simulink model "Expriment_All2"  (R2014a)
settings: Solver=FixedStepDiscrete  SolverMode=SingleTasking  StartTime=0.0  StopTime=inf  FixedStep=0.01  RelTol=1e-3
PostLoadFcn:
  | h_RPStest = RPStest;
model workspace (MAT data in the model file):
  gtest = 0
undefined symbols (not defined in the file or in its folder): avert, avert_freq_factor, avert_gaze_dirs_chance, avert_gaze_duration_factor, avert_head_frequency_factor, avert_head_speed, BML, BML1, BML2, bmlsL, bmlsM, bodyBusyFlag, clock, emotion_amount_factor, faceBusyFlag, fileID, GAZE_WIN, gazing, mut_freq_factor, mutual_gaze_duration_factor, P, pose_cat_chance, pose_chanc_factor, pose_chance_factor, pose_frequency_factor, pose_lean, pose_lean_flag, pose_speed, pose_twitch, pr, serial, STATE_BEFORE, STATE_GO, STATE_OVER, STATE_READY, Stateflow
libraries: simulink x24, instrumentlib x6, lib_affectiveChar_behavior x2, realtime_pacer_lib x2, lib_affectiveChar_input x1
(part 3 of 7)

== matlab function Expriment_All2/facialExpr/facialExprGen/forloop1/displayBMLs ==
  data: e input; l input; i input double size=1 [1..]; bml input
function fcn(e,l,i,bml)
%#codegen
fprintf('%s','e:');fprintf('%f',e);
fprintf('%s','  ,L:');fprintf('%f',l);
fprintf('%s','  ,i:');fprintf('%f',i);
disp(decArr2Str(bml));

== matlab function Expriment_All2/facialExpr/facialExprGen/forloop1/makeBmls ==
  data: i input double size=1 [1..]; arrAU input; eAmount input; arrBML output
function arrBML = fcn(i,arrAU,eAmount)
    %#codegen
    coder.extrinsic('sprintf');
    coder.extrinsic('strcat');
    
    %Maryam, 14-10-2015
    %'strcat' dimension 2  maximum size is 453,it was not possible to concat and send all bmls 
    %for one emotion together(used simulink for loop )    
    
    AU=arrAU(i);eA=eAmount(i);   
    c1 = countDigits(AU);c2 = countDigits(eA);

    str1 = sprintf('<?xml version=\"1.0\" ?><act><bml>');
    
    if(max(ceil(log10(abs(AU))),1)==1) %if AU is one-digit
        temp = sprintf('<face type=\"FACS\" side=\"BOTH\" au=\"%1d\"  start=\"0\" ready=\"1\" stroke=\"2\"  relax=\"3\" end=\"4\" amount=\"%0.1f\"/>',AU,eA); 
        temp2=strcat(str1,temp);
        str1=temp2;
    else      
        temp = sprintf('<face type=\"FACS\" side=\"BOTH\" au=\"%2d\" start=\"0\" ready=\"1\" stroke=\"2\"  relax=\"3\" end=\"4\" amount=\"%0.1f\"/>',AU,eA);
        temp2=strcat(str1,temp);
        str1=temp2;
    end

    str2 = sprintf('</bml></act>');
    %n=length(arrAU);
    %mystr=blanks(arrAU(n));
    mystr=blanks(140+c1+c2);
    mystr = strcat (str1,str2);    
    arrBML = encStr2Arr(mystr);

== matlab function Expriment_All2/EmotionSubsystem/calculateValenceArousal/HELN_VA_Emo ==
  data: V input; e output double size=1; A input double
function e = fcn(V, A)

aVarTruthTableCondition_1 = false;
aVarTruthTableCondition_2 = false;
aVarTruthTableCondition_3 = false;
aVarTruthTableCondition_4 = false;
aVarTruthTableCondition_5 = false;
aVarTruthTableCondition_6 = false;
aVarTruthTableCondition_7 = false;
aVarTruthTableCondition_8 = false;


% 7-happy  2,1

aVarTruthTableCondition_1 = logical(V>10 && A<40 && A>10);

% 8-ex  1,2 AND 2,2

aVarTruthTableCondition_2 = logical(V>0 && A>40);

% 4-fear  -1,2 AND -2,2

aVarTruthTableCondition_3 = logical(V<0 && A>40);

% 3-frust  -2,1

aVarTruthTableCondition_4 = logical(V<-10 && A<40 && A>10);

% 6-idle  2,-1

aVarTruthTableCondition_5 = logical(V>10 && A<-10 && A>-40);

% 5-calm  1,-2 AND 2,-2

aVarTruthTableCondition_6 = logical(V>0 && A<-40);

% 1-bored  -1,-2 AND -2,-2

aVarTruthTableCondition_7 = logical(V<0 && A<-40);

% 2-sad  -2,-1

aVarTruthTableCondition_8 = logical(V<-10 && A<-10 && A>-40);

if (aVarTruthTableCondition_1)
    aFcnTruthTableAction_1();
elseif (aVarTruthTableCondition_2)
    aFcnTruthTableAction_2();
elseif (aVarTruthTableCondition_3)
    aFcnTruthTableAction_3();
elseif (aVarTruthTableCondition_4)
    aFcnTruthTableAction_4();
elseif (aVarTruthTableCondition_5)
    aFcnTruthTableAction_5();
elseif (aVarTruthTableCondition_6)
    aFcnTruthTableAction_6();
elseif (aVarTruthTableCondition_7)
    aFcnTruthTableAction_7();
elseif (aVarTruthTableCondition_8)
    aFcnTruthTableAction_8();
else % Default
    aFcnTruthTableAction_5();
end

function aFcnTruthTableAction_1()

% happy

e=7;

function aFcnTruthTableAction_2()

% excited

e=8;

function aFcnTruthTableAction_3()

% fear

e=4;

function aFcnTruthTableAction_4()

% frustration

e=3;

function aFcnTruthTableAction_5()

% idle

e=6;

function aFcnTruthTableAction_6()

% contempt

e=5;

function aFcnTruthTableAction_7()

% bored

e=1;

function aFcnTruthTableAction_8()

% sad

e=2;

== stateflow chart Expriment_All2/CharacterControl/personality_Behavior_Factors ==
  state setP
    entry:
    [mutual_gaze_duration_factor, avert_gaze_duration_factor,avert_head_frequency_factor,avert_head_speed,avert_gaze_dirs_chance,avert_freq_factor,mut_freq_factor,blink_flag, blinkperiod_min,blinkperiod_max]=sharedFunc.setGazeFactors(inV,inA,personality,personalityFlag,vaFlag,gazeArray,personalityChange);
    [pose_twitch,pose_frequency_factor,pose_chanc_factor,pose_cat_chance,pose_lean,pose_speed,pose_space,pose_lean_flag]=sharedFunc.setPoseFactors(inV,inA,personality,personalityFlag,vaFlag,poseArray,personalityChange);
  state init
    entry: mutual_gaze_duration_factor=1;avert_gaze_duration_factor=1;,avert_freq_factor=1;mut_freq_factor=1;
    avert_head_frequency_factor=20;avert_head_speed=1;avert_gaze_dirs_chance=1;blink_flag=0; blinkperiod_min=5;blinkperiod_max=9;
    pose_lean_flag=0; pose_frequency_factor=40;pose_chanc_factor=1;pose_cat_chance=50;pose_lean=18;pose_speed=1;pose_space=0;
  state wait
  state sharedFunc [group]
  (default) -> init
  init -> wait
  setP -> wait
  wait -> setP : [personalityChange==1]
  data: inA input double size=1; inV input double size=1; vaFlag input boolean size=1; personalityFlag input boolean size=1; gazeArray input double size=[1, 6]; personality input double size=1; personalityChange input boolean size=1; mutual_gaze_duration_factor data_store_memory; avert_head_frequency_factor data_store_memory; avert_gaze_duration_factor data_store_memory; avert_head_speed data_store_memory; avert_gaze_dirs_chance data_store_memory; poseArray input double size=[1, 6]; pose_chanc_factor data_store_memory; pose_frequency_factor data_store_memory; pose_lean data_store_memory; pose_change_flag data_store_memory; pose_lean_flag data_store_memory; pose_speed data_store_memory; pose_cat_chance data_store_memory; internalE input double size=1; emotion_amount_custom input double size=1; emotion_amount_factor data_store_memory size=1; mut_freq_factor data_store_memory; avert_freq_factor data_store_memory; pose_twitch data_store_memory; blinkperiod_min data_store_memory; blink_flag data_store_memory; blinkperiod_max data_store_memory; pose_space data_store_memory

== stateflow chart Expriment_All2/CharacterControl/custom_Behavior_Factors ==
  state setP
    entry:
    [mutual_gaze_duration_factor, avert_gaze_duration_factor,avert_head_frequency_factor,avert_head_speed,avert_gaze_dirs_chance,avert_freq_factor,mut_freq_factor]=sharedFunc.setGazeFactors(inV,inA,personality,personalityFlag,vaFlag,gazeArray,personalityChange);
  state init
    entry: mutual_gaze_duration_factor=1;avert_gaze_duration_factor=1;
    avert_head_frequency_factor=1;avert_head_speed=1;avert_gaze_dirs_chance=1;,avert_freq_factor=1;mut_freq_factor=1;
    pose_frequency_factor=5;pose_chanc_factor=1;pose_cat_chance=10;pose_lean=10;pose_speed=1;pose_lean_flag=0;
  state wait
  state sharedFunc [group]
  state setP1
    entry:
    [pose_twitch,pose_frequency_factor,pose_chanc_factor,pose_cat_chance,pose_lean,pose_speed,pose_lean_flag]=sharedFunc.setPoseFactors(inV,inA,personality,personalityFlag,vaFlag,poseArray,personalityChange);
  (default) -> init
  wait -> setP [order 1] : [gazeArray(:,1)==1]
  setP -> wait
  init -> wait
  setP1 -> wait
  wait -> setP1 [order 2] : [poseArray(:,1)==1]
  data: inA input double size=1; inV input double size=1; vaFlag input boolean size=1; personalityFlag input boolean size=1; gazeArray input double size=[1, 6]; personality input double size=1; personalityChange input boolean size=1; mutual_gaze_duration_factor data_store_memory; avert_head_frequency_factor data_store_memory; avert_gaze_duration_factor data_store_memory; avert_head_speed data_store_memory; avert_gaze_dirs_chance data_store_memory; poseArray input double size=[1, 6]; pose_lean data_store_memory; pose_speed data_store_memory; pose_chanc_factor data_store_memory; pose_frequency_factor data_store_memory; pose_cat_chance data_store_memory; pose_lean_flag data_store_memory; emotion_amount_custom input double size=1; emotion_amount_factor data_store_memory size=1; mut_freq_factor data_store_memory; avert_freq_factor data_store_memory; pose_twitch data_store_memory

== matlab function Expriment_All2/EmotionSubsystem/calculateValenceArousal/HELN plot ==
  data: v input; a input
function fcn(v,a)
%coder.extrinsic to bypass code generation
coder.extrinsic('fscanf')
coder.extrinsic('get_param');
% coder.extrinsic('importdata');

currentTime=get_param('Expriment_FacialExpr','SimulationTime');%use name of simulink proj

A = [v;a;currentTime];

fileID = fopen('HELN_VA_table.txt','a');
fprintf(fileID,'%0.1f,%0.1f,%0.1f\r\n',A);
fclose(fileID);

%use the following to draw the plot
%tmp_data = importdata('HEHN_VA_table.txt',','); 
%no need: x=tmp_data(:,1);y=tmp_data(:,2);z=tmp_data(:,3)
%matrix=tmp_data
%tri = delaunay(matrix(:,1),matrix(:,2));
%trisurf(tri,matrix(:,1),matrix(:,2),matrix(:,3))
%shading interp

%-----------------------------------------
% fileID = fopen('HEHN_VA_table.txt','r');
% formatSpec = '%1f\r %1f\r %1f\r\n';
% sizeA = [3 Inf];
% A = fscanf(fileID,formatSpec,sizeA)
% % A = A'
% fclose(fileID);

% x = zeros(100,2);y = zeros(100,2);
% filename = 'HEHN_VA_table.txt';
% delimiterIn = ' ';
% headerlinesIn = 1;
% A = importdata(filename,delimiterIn,headerlinesIn);

% fileID=fopen('HEHN_VA_table4.txt');
% s=textscan(fileID,'%d %d %d','headerlines',23);
% fclose(fileID);
% x=s{1}

== matlab function Expriment_All2/EmotionSubsystem/calculateValenceArousal/HEHN_V ==
  data: v2 output double size=1; v1 input double size=1
function v2 = fcn(v1)

aVarTruthTableCondition_1 = false;
aVarTruthTableCondition_2 = false;



aVarTruthTableCondition_1 = logical(v1>10);


aVarTruthTableCondition_2 = logical(v1<-10);

if (aVarTruthTableCondition_1)
    aFcnTruthTableAction_1();
elseif (aVarTruthTableCondition_2)
    aFcnTruthTableAction_2();
else % Default
    aFcnTruthTableAction_3();
end

function aFcnTruthTableAction_1()


v2=v1;

function aFcnTruthTableAction_2()


v2=v1;

function aFcnTruthTableAction_3()


v2=0;

== matlab function Expriment_All2/EmotionSubsystem/calculateValenceArousal/LEHN_V ==
  data: v2 output double size=1; v1 input double size=1
function v2 = fcn(v1)

aVarTruthTableCondition_1 = false;
aVarTruthTableCondition_2 = false;



aVarTruthTableCondition_1 = logical(v1>25);


aVarTruthTableCondition_2 = logical(v1<-25);

if (aVarTruthTableCondition_1)
    aFcnTruthTableAction_1();
elseif (aVarTruthTableCondition_2)
    aFcnTruthTableAction_2();
else % Default
    aFcnTruthTableAction_3();
end

function aFcnTruthTableAction_1()


v2=v1;

function aFcnTruthTableAction_2()


v2=v1;

function aFcnTruthTableAction_3()


v2=0;

== matlab function Expriment_All2/EmotionSubsystem/calculateValenceArousal/LELN_A ==
  data: a2 output double size=1; a1 input double size=1
function a2 = fcn(a1)

aVarTruthTableCondition_1 = false;
aVarTruthTableCondition_2 = false;



aVarTruthTableCondition_1 = logical(a1>25);


aVarTruthTableCondition_2 = logical(a1<-25);

if (aVarTruthTableCondition_1)
    aFcnTruthTableAction_1();
elseif (aVarTruthTableCondition_2)
    aFcnTruthTableAction_2();
else % Default
    aFcnTruthTableAction_3();
end

function aFcnTruthTableAction_1()


a2=a1;

function aFcnTruthTableAction_2()


a2=a1;

function aFcnTruthTableAction_3()


a2=0;

== matlab function Expriment_All2/EmotionSubsystem/calculateValenceArousal/LELN_VA_Emo ==
  data: V input; e output double size=1; A input double
function e = fcn(V, A)

aVarTruthTableCondition_1 = false;
aVarTruthTableCondition_2 = false;
aVarTruthTableCondition_3 = false;
aVarTruthTableCondition_4 = false;
aVarTruthTableCondition_5 = false;
aVarTruthTableCondition_6 = false;
aVarTruthTableCondition_7 = false;
aVarTruthTableCondition_8 = false;


% 7-happy  2,1

aVarTruthTableCondition_1 = logical(V>20 && A<40 && A>20);

% 8-ex  1,2 AND 2,2

aVarTruthTableCondition_2 = logical(V>0 && A>40);

% 4-fear  -1,2 AND -2,2

aVarTruthTableCondition_3 = logical(V<0 && A>40);

% 3-frust  -2,1

aVarTruthTableCondition_4 = logical(V<-20 && A<40 && A>20);

% 6-idle  2,-1

aVarTruthTableCondition_5 = logical(V>20 && A<-20 && A>-40);

% 5-calm  1,-2 AND 2,-2

aVarTruthTableCondition_6 = logical(V>0 && A<-40);

% 1-bored  -1,-2 AND -2,-2

aVarTruthTableCondition_7 = logical(V<0 && A<-40);

% 2-sad  -2,-1

aVarTruthTableCondition_8 = logical(V<-20 && A<-20 && A>-40);

if (aVarTruthTableCondition_1)
    aFcnTruthTableAction_1();
elseif (aVarTruthTableCondition_2)
    aFcnTruthTableAction_2();
elseif (aVarTruthTableCondition_3)
    aFcnTruthTableAction_3();
elseif (aVarTruthTableCondition_4)
    aFcnTruthTableAction_4();
elseif (aVarTruthTableCondition_5)
    aFcnTruthTableAction_5();
elseif (aVarTruthTableCondition_6)
    aFcnTruthTableAction_6();
elseif (aVarTruthTableCondition_7)
    aFcnTruthTableAction_7();
elseif (aVarTruthTableCondition_8)
    aFcnTruthTableAction_8();
else % Default
    aFcnTruthTableAction_5();
end

function aFcnTruthTableAction_1()

% happy

e=7;

function aFcnTruthTableAction_2()

% excited

e=8;

function aFcnTruthTableAction_3()

% fear

e=4;

function aFcnTruthTableAction_4()

% frustration

e=3;

function aFcnTruthTableAction_5()

% idle

e=6;

function aFcnTruthTableAction_6()

% contempt

e=5;

function aFcnTruthTableAction_7()

% bored

e=1;

function aFcnTruthTableAction_8()

% sad

e=2;

== matlab function Expriment_All2/EmotionSubsystem/satFunction ==
  data: randv input; smile input; wave input; win input; invade input; v_trigW output; vaFlag input; v_trig output
function [v_trigW,v_trig]= fcn(randv,smile,wave,win,invade,vaFlag)
%#codegen
% 30/06/2015
    %Here set Agent's satisfaction flag based on your scenario
    %In RPS scenario agent gets satisfined when she wins. states of interaction= {STATE_READY=7;
    %STATE_GO=1;STATE_HAND=2;STATE_OVER=3; STATE_BEFORE=4;STATE_RESULT=5;STATE_WAIT=6;}
   
    if(vaFlag==1)
        v_trigW=0;%weight by which valence value is changed (sum of weight of all triggers)
        %randv 30% chance of random increase or decrease in valence
        randTrigger=floor(randv);
        if(0<randTrigger)&&(randTrigger<30)
            v_trigW = v_trigW + 0.6;
        end
        if(30<randTrigger)&&(randTrigger<60)
            v_trigW = v_trigW - 0.6;
        end

        if(win==2) %agent wins so she is satisfied
            v_trigW = v_trigW + 0.5;
        elseif(win==1) %user wins so agent is NOT satisfied
            v_trigW = v_trigW - 0.5;
        end

        if(smile==1)
            v_trigW=v_trigW+0.25;
        end

        if(wave==1)
            v_trigW=v_trigW+0.25;
        end

        if(invade==1)
            v_trigW=v_trigW-0.25;
        end
    else
         v_trigW=0;
    end
    if(v_trigW>0)
        v_trig=1;
    elseif(v_trigW<0)
        v_trig=-1;
        v_trigW=abs(v_trigW);
    else
        v_trig=0;
    end

== matlab function Expriment_All2/CharacterControl/personality_Behavior_Factors/sharedFunc ==
  data: v function_input double size=1; a function_input double size=1; mutDurFactor function_output double size=1; avertDurFactor function_output double size=1; avertHeadFreqFactor function_output double size=1; p function_input double size=1; pFlag function_input boolean size=1; vaFlag function_input boolean size=1; avertHeadSpeed function_output double size=1; gazeArr function_input double size=[1,6]; avertDirsChance function_output double size=1; avertFreqFactor function_output double size=1; mutFreqFactor function_output double size=1; blinkFlag function_output double size=1; blinkPeriodMin function_output double size=1; blinkPeriodMax function_output double size=1; personalityChange function_input double size=1; poseTwitch function_output double size=1; poseFreqFactor function_output double size=1; poseChanceFactor function_output double size=1; poseCatChance function_output double size=1; poseLean function_output double size=1; v function_input double size=1; ar function_input double size=1; p function_input double size=1; pFlag function_input boolean size=1; vaFlag function_input boolean size=1; poseSpeed function_output double size=1; poseSpace function_output double size=1; poseArr function_input double size=[1,6]; poseLeanFlag function_output double size=1; personalityChange function_input double size=1
function [mutDurFactor,avertDurFactor,avertHeadFreqFactor,avertHeadSpeed,avertDirsChance,avertFreqFactor,mutFreqFactor,blinkFlag,blinkPeriodMin,blinkPeriodMax]=setGazeFactors(v,a,p,pFlag,vaFlag,gazeArr,personalityChange)
    % Valence/Arousal: ref?
    %V+A+ (excite,happy):high mutual dur,head avert freq less,high freq of change btw mut/avert(MMMMMMMAAMMMMMAMMMA)
    %V-A+ (fear,frust): mid mut/avert,,head avert freq mid,high freq of change btw mut/avert(MMAAMMMAAMMAAAMMMAAAMA)
    %V+A- (idle, calm): mid mut/avert,head avert freq mid,low freq of change btw mut/avert(MMMMMMMAAAAAAMMMMMAAAAA)
    %V-A- (bored,sad):  avert dur more,,head avert freq more,,high freq of change btw mut/avert(AAAAAAMAAAAAAAAMAAAAA)
    %V+A+: v>0 & a>0,V-A+: v<0 & a>0,V+A-:v>0 & a<0,V-A-:v<0 & a<0

    %paper: Effects of Direct and Averted Gaze on the Perception of Facially Communicated Emotion
    % rate of approach-oriented dispositions (i.e., anger and joy) higher for direct relative gaze stimuli
    %avoidance-oriented dispositions (i.e., fear and sadness) would be higher for averted gaze faces.

    %russel, mehrabian circumplex:
    % v-mid,a-mid:approach;     v-mid,a+:avoid;       v-mid,a-:avoid
    % v+,a-mid:mid-approach;    v+,a+:high-approach;  v+,a-:low-approach
    % v-,a-mid:mid-avoid;        v-,a+:high-avoid;    v-,a-:low-avoid

    % marsella, emotional gaze:
    % a+:high blink, faster move
    
    %PERSONALITY:
    % HEHN:mutual dur more,head avert freq more,high freq of change btw mut/avert(MAMAMMAMMMAMAMMAMMAMA)
    % LEHN:avert dur  more,head avert freq more, high freq of change btw mut/avert(AMAAMAAAMAMAAAMAAMAAM)
    % HELN:mutual dur  more,head avert freq less,low freq of change btw mut/avert(MMMMMMMAMMMMMMMMAMMM)
    % LELN:avert  dur more,head avert freq more,low freq of change btw mut/avert(AAAAAAMAAAAAAAAMAAAAA)
    
    %Perception of personality through eye gaze, Ruhland et al
    %Extravert: gaze tward,long,often,up-center-left-right; few blinks ; wide fast node
    %Introvert: gaze Avoidance,short,seldom,down-center; normal blinks; small slow node
    %Neurotic: gaze Avoidance,short,seldom,down-left-right; often blinks; None
    %Stable: gaze tward,medium,medium,center-left-right; normal blinks ; None
    
    %Saccadic reaction time is between 0.18sec and 0.22sec on average.Minimum intersaccadic interval ranges from 0.05sec to 0.1sec
    %smartbody DOF:magnitude:~btw 5'&12'->chanceO:btw 3&8->aveDur:btw 0.26sec&0.18sec --> 
    %simulation sample time is 0.001 so btw 26 and 18
    %magnitude=-6.9*log(chanceO/15.7) -->  -6.9*log(3/15.7)=11.4,-6.9*log(8/15.7)=4.6
    %chanceO=randArray(:,7)-->(3,8); 
    %avertDur=(25+2.5*magnitude)/2*factor;(same for mutual):btw(25+2.5*11.4)/2=26,(25+2.5*4.6)/2=18
    %randHeadChance=randi([1,1+round(randArray(3,5)/avert_head_frequency_factor)]);

    mutDurFactor=1; 
    avertDurFactor=1;  
    avertHeadFreqFactor=20;
    avertHeadSpeed=1;%1=normal, 2=fast&up,3=slow&down
    avertDirsChance=0;%not 1 & 2 is normal
    avertFreqFactor=1;
    mutFreqFactor=1;
    blinkFlag=0;
    blinkPeriodMin=5.0; %normal
    blinkPeriodMax=9.0;%normal

    if(pFlag==1)
        if(personalityChange==1)
            blinkFlag=1;disp('personality changed.');
        end
        if(p==1)%HEHN  
            mutDurFactor=2; % HEHN mut longer ,((25+2.5*magnitude)*mutual_gaze_duration_factor)/7;
            avertDurFactor=0.5;%HE avert short,3' to 4',btw (25+2.5*magnitude)*avert_gaze_duration_factor)/7;
            mutFreqFactor=4;%HE mut long,12' to 17'
            avertFreqFactor=0.25;% val/4, HE avert gaze low
            
            avertHeadFreqFactor=30;%HE often head,[avert_head_frequency_factor>randrandi(0,100)]
            avertHeadSpeed=2;%HE fast&up, headSpeed={1,2,3}
            avertDirsChance=1;%HE up            
            
            blinkPeriodMin=0.15; %HN often blinks
            blinkPeriodMax=6.0;%HE few blinks
        elseif(p==2) %LEHN %LE normal blinks, HN often blinks
            mutDurFactor=0.5; % LE mut less(mutDur/10) ,HN freq more
            avertDurFactor=2; % (avertDur/4)
            mutFreqFactor=0.15;
            avertFreqFactor=4;
            
            avertHeadFreqFactor=15;%LE avert low
            avertHeadSpeed=3;%LE slow&down
            avertDirsChance=2;%LE down
           
            blinkPeriodMin=0.2; %often
            blinkPeriodMax=5.0;%norm
        elseif(p==3) %HELN %HE few blinks, LN normal blinks 
            mutDurFactor=4; % HE dur more, LN freq less
            avertDurFactor=0.1; % /4 
            mutFreqFactor=4;
            avertFreqFactor=0.25;
            
            avertHeadFreqFactor=25;%HE avert head more
            avertHeadSpeed=2;%fast&up
            avertDirsChance=1;%HE up            
            
            blinkPeriodMin=5.0; %normal
            blinkPeriodMax=15.0;%few
        else %LELN %LE normal blinks, LN normal blinks 
            mutDurFactor=0.25; % /4 
            avertDurFactor=0.5;% /2 
            mutFreqFactor=0.25;
            avertFreqFactor=4;
            
            avertHeadFreqFactor=10;%LE avert head less
            avertHeadSpeed=3;%slow&down
            avertDirsChance=2;%LE down
          
            blinkPeriodMin=5.0; %normal
            blinkPeriodMax=9.0;%normal
        end  
    end
  
    %for emotion I should, seperate that from the controllers so they
    %calculate the depented parameters in parallel, in order to avoid a lot
    %of BMLs the checking state is repeating every 20 secs and if the value
    %is changed it sends the BML, here instead of constant value I should
    %make all of the parametric so when V & A increase or decrease it
    %affects the blink mut and avert ..
    if(vaFlag==1)
        if(v>40 && a>40)%V+A+,high-approach,mutual alot
            mutDurFactor=mutDurFactor*2; % /2
            avertDurFactor=round(avertDurFactor*0.5);  % /2
            avertHeadFreqFactor=round(avertHeadFreqFactor/3);%high-approach:head not avert
            %avertHeadSpeed=2;%aroused fast, removed ths since fast&up is together, also it makes it hard for evaluateion
            
            %27-12-2015- Best way to set the blink period is as a linear function of arousal amount
            %      val/(1+((2-1)*(A/100))) 
            %in which val is BlinkMin or BlinkMax and A is arousal amount; this function sets the
            %blinkPriodMin and max to half for twice blink in arousal=100 and to their default at 
            %arousal=1 sicne we need to re-calculate and send sbms continiously I avoided that for 
            % now, instead I only increase min and max when Arousal passes 50 threshold
            blinkPeriodMin=blinkPeriodMin/1.5; %often
            blinkPeriodMax=blinkPeriodMax/1.5;
            blinkFlag=1;
            disp(mutDurFactor);
        elseif(v<-40 && a>40) %V-A+,high-avoid, avert alot
            mutDurFactor=round(mutDurFactor*0.5); % /2
            avertDurFactor=avertDurFactor*2; % /2
            avertHeadFreqFactor=avertHeadFreqFactor+30;%high-avoid:head avert alot
            %avertHeadSpeed=2;%fast
            blinkPeriodMin=blinkPeriodMin/1.5; %often
            blinkPeriodMax=blinkPeriodMax/1.5;
            blinkFlag=1;
        elseif(v>40 && a<-40) %V+A- ,low-approach, mutual most
            mutDurFactor=round(mutDurFactor*1.5); %  /2
            avertDurFactor=round(avertDurFactor*0.75); %/2
            avertHeadFreqFactor=round(avertHeadFreqFactor/2);%approach:head not avert
            %avertHeadSpeed=1;%slow&down
            blinkFlag=0;
        elseif(v<-40 && a<-40) %V-A-,  low-avoid, avert most
            mutDurFactor=round(mutDurFactor*0.75); %/2
            avertDurFactor=round(avertDurFactor*1.5);% /2
            avertHeadFreqFactor=avertHeadFreqFactor+20;%avoid:head avert alot
            %avertHeadSpeed=1;%slow&down, if he is extrovert we dont want him to look down even if low aroused
            blinkFlag=0;
        end  
    end

== matlab function Expriment_All2/CharacterControl/personality_Behavior_Factors/sharedFunc ==
function [poseTwitch,poseFreqFactor,poseChanceFactor,poseCatChance,poseLean,poseSpeed,poseSpace,poseLeanFlag]=setPoseFactors(v,ar,p,pFlag,vaFlag,poseArr,personalityChange)   
    
    pose_custom_flag=poseArr(:,1);
    pose_chance_custom=poseArr(:,3);
    pose_selfAdaptor_chance_custom=poseArr(:,2);
    pose_frequency_custom=poseArr(:,4);
    pose_speed_custom=poseArr(:,5);
    pose_lean_custom=poseArr(:,6);

    poseCatChance=50;%defalut 50% chance of selfA or weightShift, due low num of weightShift
    poseChanceFactor=1;%if (not similar duration btw poses always)
    poseFreqFactor=40;
    poseSpeed=1;%1=normal;2=fast; 3=slow;
    poseLean=18;
    poseTwitch=0;
    poseLeanFlag=0;
    poseSpace=0;% normal people dont do spacious gestures

    if(pose_custom_flag==0)    
        if(pFlag==1)
            if(personalityChange==1)
                poseLeanFlag=1;
            end
            if(p==1) %HEHN
                 poseTwitch=1;%HN
                 poseFreqFactor=15;%HN more freq,after(pose_frequency_factor,secs)
                 poseLean=18;
                 poseChanceFactor=4;% HN high chance,randPoseChance=randi([0,round(interest*randSlowPose/pose_chance_factor)]);
                 poseCatChance=90;%HN high selfA,[randPR<=pose_selfAdaptor_chance_factor ]
                 poseSpeed=2;%HE fast
                 %poseSpace=1;%HE
             elseif(p==2)%LEHN
                 poseTwitch=1;%HN
                 poseFreqFactor=20;%HN more freq but low speed
                 poseLean=19;
                 poseChanceFactor=4;%HN high chance
                 poseCatChance=10;%HN high:90% adaptor
                 poseSpeed=3;%LE slow
                 %poseSpace=0;%LE
             elseif(p==3)%HELN
                 poseTwitch=0;%LN
                 poseFreqFactor=50;%LN low chance
                 poseLean=18;
                 poseChanceFactor=1;%LN low chance
                 poseCatChance=10;%  10% adapter
                 poseSpeed=2;%HE
                 %poseSpace=1;%HE
             elseif(p==4)%LELN
                 poseTwitch=0;%LN
                 poseFreqFactor=60;%LE
                 poseLean=19;
                 poseChanceFactor=1;%LN low chance
                 poseCatChance=90;
                 poseSpeed=3;%LE
                 %poseSpace=0;%LE
            else%no personality, its should not come here
                fprintf(' Error: the personality is not listed, back to normal, p=: '); fprintf('%0.0f',p);
                poseCatChance=70;
                poseChanceFactor=1;
                poseFreqFactor=40;
                poseSpeed=1;%1=normal;2=fast; 3=slow;
                poseLean=18;
                poseTwitch=0;
                poseLeanFlag=0;
                poseSpace=0;% normal people dont do spacious gestures
             end
        end
%     29-12-2015  I removed this since it intefere with personality's effect on pose
%     % marsella, emotional gaze:
%     % a+:faster move,body fw
%     if(vaFlag==1)
%         if( ar>50)%A+
%              poseSpeed=2;%high arouse fast move
%              poseLeanFlag=12;%high aroused lean fw
%         end
%         if(ar<-50)%A-
%              poseSpeed=3;%low arouse slow move
%              poseLeanFlag=11;%low aroused lean back
%         end
%     end 
    
    else%custom-flag==1
        poseFreqFactor=pose_frequency_custom;
        poseLean=pose_lean_custom;
        poseChanceFactor=pose_chance_custom;
        poseCatChance=pose_selfAdaptor_chance_custom;
        poseSpeed=pose_speed_custom;
    end

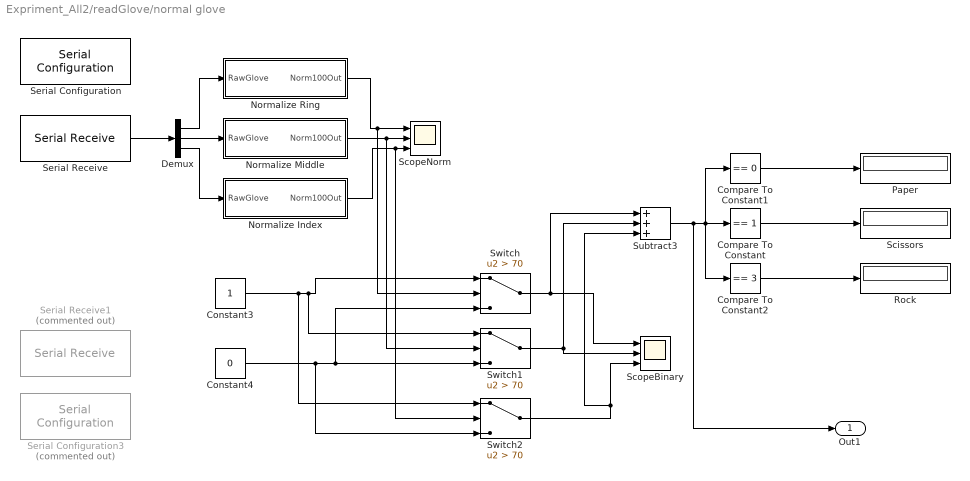
== system Expriment_All2/readGlove/normal glove ==
  Compare To Constant : simulink/Logic and Bit Operations/Compare To Constant  relop===  const=1  OutDataTypeStr=boolean
  Compare To Constant1 : simulink/Logic and Bit Operations/Compare To Constant  relop===  const=0  OutDataTypeStr=boolean
  Compare To Constant2 : simulink/Logic and Bit Operations/Compare To Constant  relop===  const=3  OutDataTypeStr=boolean
  Constant3 : Constant
  Constant4 : Constant  Value=0
  Demux : Demux  Outputs=3
  Normalize Index : Subsystem
  Normalize Middle : Subsystem
  Normalize Ring : Subsystem
  Paper : Display
  Rock : Display
  Scissors : Display
  ScopeBinary : Scope  NumInputPorts=3
      settings: YMin=-0.5~-0.5~-0.5  YMax=1.5~1.5~1.5
  ScopeNorm : Scope  NumInputPorts=3
      settings: TimeRange=10  YMin=-20~-20~-20  YMax=150~150~150
  Serial Configuration : instrumentlib/Serial Configuration  Priority=-200000  ComPortMenu=<Please select a port...>  ComPort=COM4  ObjConstructor=serial('COM4');  BaudRate=9600  DataBits=8  Parity=none  StopBits=1  FlowControl=none  Timeout=10  ByteOrder=LittleEndian
  Serial Configuration3 : instrumentlib/Serial Configuration  Priority=-200000  Commented=on  ComPortMenu=<Please select a port...>  ComPort=COM5  ObjConstructor=serial('COM5');  BaudRate=9600  DataBits=8  Parity=none  StopBits=1  FlowControl=none  Timeout=10  ByteOrder=LittleEndian
  Serial Receive : instrumentlib/Serial Receive  ComPortMenu=<Please select a port...>  ComPort=COM4  ObjConstructor=serial('COM4');  Terminator=<none>  DataSize="[3  1]"  DataType=uint8  EnableBlockingMode=on  ActionDataUnavailable=Output last received value  CustomValue=0  SampleTime=0.01
  Serial Receive1 : instrumentlib/Serial Receive  Commented=on  ComPortMenu=<Please select a port...>  ComPort=COM5  ObjConstructor=serial('COM5');  Terminator=<none>  DataSize="[3  1]"  DataType=uint8  EnableBlockingMode=on  ActionDataUnavailable=Output last received value  CustomValue=0  SampleTime=0.01
  Subtract3 : Sum  Inputs=+++
  Switch : Switch  Criteria=u2 > Threshold  Threshold=70
  Switch1 : Switch  Criteria=u2 > Threshold  Threshold=70
  Switch2 : Switch  Criteria=u2 > Threshold  Threshold=70
  Out1 : Outport
  wires:
  Demux/1 -> Normalize Ring/1(RawGlove)
  Demux/2 -> Normalize Middle/1(RawGlove)
  Demux/3 -> Normalize Index/1(RawGlove)
  Switch/1 -> ScopeBinary/1, Subtract3/1
  Constant3/1 -> Switch2/1, Switch1/1, Switch/1
  Constant4/1 -> Switch2/3, Switch1/3, Switch/3
  Switch1/1 -> ScopeBinary/2, Subtract3/2
  Switch2/1 -> Subtract3/3, ScopeBinary/3
  Subtract3/1 -> Compare To Constant/1, Compare To Constant2/1, Compare To Constant1/1, Out1/1
  Compare To Constant1/1 -> Paper/1
  Compare To Constant/1 -> Scissors/1
  Compare To Constant2/1 -> Rock/1
  Normalize Index/1(Norm100Out) -> Switch2/2, ScopeNorm/3
  Normalize Ring/1(Norm100Out) -> Switch/2, ScopeNorm/1
  Normalize Middle/1(Norm100Out) -> ScopeNorm/2, Switch1/2
  Serial Receive/1 -> Demux/1

== system Expriment_All2/readSHORE/smile ==
  In1 : Inport
  ifSmile : MATLAB Function  TreatAsAtomicUnit=on
  Out1 : Outport
  wires:
  ifSmile/1(y) -> Out1/1
  In1/1 -> ifSmile/1(u)

== system Expriment_All2/GazeFollowSubsystem/reactiveGaze/createGazePawn/sendBML ==
  In1 : Inport  OutDataTypeStr=double  PortDimensions=[1000 1]
  f : TriggerPort  TriggerType=function-call
      settings: CopyFcn=Stateflow.SLINSF.SimulinkMan.removeBlockPreDeleteFcn  PreDeleteFcn=Stateflow.SLINSF.SimulinkMan.unsafePredeleteFcn
  C++ S-Function2 : S-Function  FunctionName=yarpSendText_sfun  Parameters='/sim/out/bml8', '/SB/in/bml'  EnableBusSupport=off
  wires:
  In1/1 -> C++ S-Function2/1

== system Expriment_All2/GazeFollowSubsystem/reactiveGaze/createGazePawn/sendSBM ==
  In2 : Inport  OutDataTypeStr=double  PortDimensions=[1000 1]
  f : TriggerPort  TriggerType=function-call
      settings: CopyFcn=Stateflow.SLINSF.SimulinkMan.removeBlockPreDeleteFcn  PreDeleteFcn=Stateflow.SLINSF.SimulinkMan.unsafePredeleteFcn
  C++ S-Function2 : S-Function  FunctionName=yarpSendText_sfun  Parameters='/sim/out/smb5', '/SB/in/sbm'  EnableBusSupport=off
  wires:
  In2/1 -> C++ S-Function2/1

== system Expriment_All2/GazeFollowSubsystem/reactiveGaze/reactiveGazeControl ==
  x : Inport
  y : Inport  Port=2
  C++ S-Function2 : S-Function  FunctionName=yarpSendText_sfun  Parameters='/sim/out/smb7', '/SB/in/sbm'  EnableBusSupport=off
  reactiveMovePawn : MATLAB Function  TreatAsAtomicUnit=on
  wires:
  x/1 -> reactiveMovePawn/1(x)
  y/1 -> reactiveMovePawn/2(y)
  reactiveMovePawn/1(arrBML) -> C++ S-Function2/1

== system Expriment_All2/GazeFollowSubsystem/resetGazeTarget/createGazePawn/sendSBM ==
  In2 : Inport  OutDataTypeStr=double  PortDimensions=[1000 1]
  f : TriggerPort  TriggerType=function-call
      settings: CopyFcn=Stateflow.SLINSF.SimulinkMan.removeBlockPreDeleteFcn  PreDeleteFcn=Stateflow.SLINSF.SimulinkMan.unsafePredeleteFcn
  C++ S-Function2 : S-Function  FunctionName=yarpSendText_sfun  Parameters='/sim/out/smb8', '/SB/in/sbm'  EnableBusSupport=off
  wires:
  In2/1 -> C++ S-Function2/1

== system Expriment_All2/facialExpr/facialExprGen/emotionBMLsLoop ==
  Amounts : Inport
  AUs : Inport  Port=2
  i : Inport  Port=3  OutMin=1  OutDataTypeStr=double
  e : Inport  Port=4
  Delay : Delay  DelayLength=10  InitialCondition=10
  For Iterator : ForIterator  IterationSource=external
  bml1 : M-S-Function  FunctionName=yarpSendText2_sfun  Parameters='/sim/out/bml9', '/SB/in/bml'
  displayBMLs : MATLAB Function  TreatAsAtomicUnit=on
  loopInBmls : MATLAB Function  TreatAsAtomicUnit=on
  wires:
  AUs/1 -> loopInBmls/2(arrAU)
  Amounts/1 -> loopInBmls/3(eAmount)
  loopInBmls/1(arrBML) -> Delay/1, displayBMLs/3(bml)
  e/1 -> displayBMLs/1(e)
  Delay/1 -> bml1/1
  i/1 -> loopInBmls/1(i), displayBMLs/2(i)

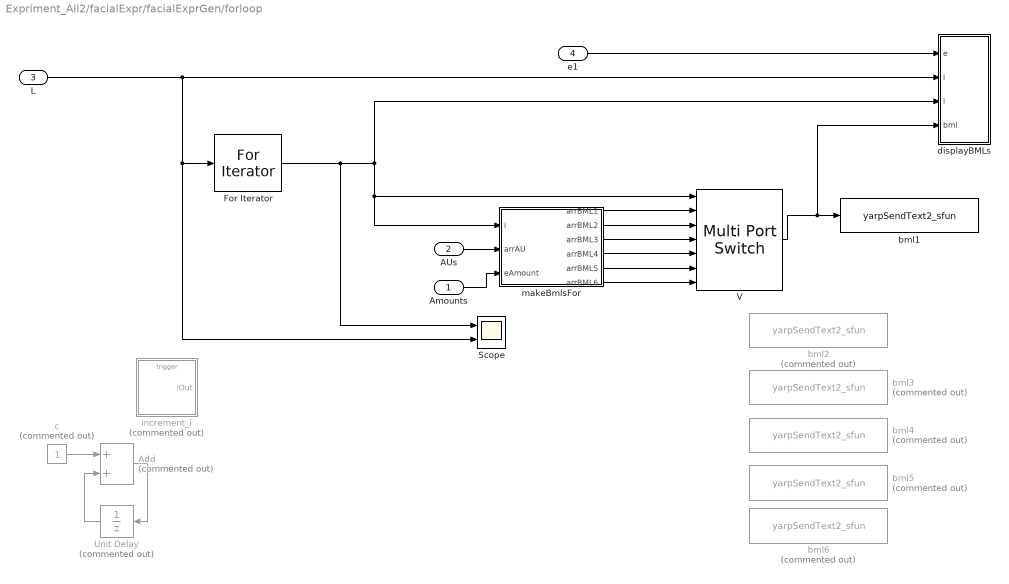
== system Expriment_All2/facialExpr/facialExprGen/forloop ==
  Amounts : Inport
  AUs : Inport  Port=2
  L : Inport  Port=3
  e1 : Inport  Port=4
  Add : Sum  Commented=on
  For Iterator : ForIterator  IterationSource=external  IterationVariableDataType=double
  Scope : Scope  NumInputPorts=2
      settings: YMin=3~3  YMax=3~3  SaveName=ScopeData7
  Unit Delay : UnitDelay  Commented=on  SampleTime=0.01
  V : MultiPortSwitch  Inputs=6
  bml1 : M-S-Function  FunctionName=yarpSendText2_sfun  Parameters='/sim/out/bml9', '/SB/in/bml'
  bml2 : M-S-Function  Commented=on  FunctionName=yarpSendText2_sfun  Parameters='/sim/out/bml10', '/SB/in/bml'
  bml3 : M-S-Function  Commented=on  FunctionName=yarpSendText2_sfun  Parameters='/sim/out/bml11', '/SB/in/bml'
  bml4 : M-S-Function  Commented=on  FunctionName=yarpSendText2_sfun  Parameters='/sim/out/bml12', '/SB/in/bml'
  bml5 : M-S-Function  Commented=on  FunctionName=yarpSendText2_sfun  Parameters='/sim/out/bml13', '/SB/in/bml'
  bml6 : M-S-Function  Commented=on  FunctionName=yarpSendText2_sfun  Parameters='/sim/out/bml14', '/SB/in/bml'
  c : Constant  Commented=on
  displayBMLs : MATLAB Function  TreatAsAtomicUnit=on
  increment_i : Subsystem  Commented=on
  makeBmlsFor : MATLAB Function  TreatAsAtomicUnit=on
  wires:
  L/1 -> Scope/2, For Iterator/1, displayBMLs/2(l)
  AUs/1 -> makeBmlsFor/2(arrAU)
  Amounts/1 -> makeBmlsFor/3(eAmount)
  e1/1 -> displayBMLs/1(e)
  Unit Delay/1 -> Add/2
  c/1 -> Add/1
  Add/1 -> Unit Delay/1
  For Iterator/1 -> Scope/1, V/1, makeBmlsFor/1(i), displayBMLs/3(i)
  V/1 -> displayBMLs/4(bml), bml1/1
  makeBmlsFor/1(arrBML1) -> V/2
  makeBmlsFor/2(arrBML2) -> V/3
  makeBmlsFor/3(arrBML3) -> V/4
  makeBmlsFor/4(arrBML4) -> V/5
  makeBmlsFor/5(arrBML5) -> V/6
  makeBmlsFor/6(arrBML6) -> V/7

== system Expriment_All2/facialExpr/facialExprGen/forloop1 ==
  Amounts : Inport
  AUs : Inport  Port=2
  L : Inport  Port=3
  e1 : Inport  Port=4
  Add : Sum  Commented=on
  Delay : Delay  DelayLength=50  InitialCondition=0
  For Iterator : ForIterator  IterationSource=external  IterationVariableDataType=double
  Scope : Scope  NumInputPorts=2
      settings: YMin=3~3  YMax=3~3  SaveName=ScopeData7
  Unit Delay : UnitDelay  Commented=on  SampleTime=0.01
  bml1 : M-S-Function  FunctionName=yarpSendText2_sfun  Parameters='/sim/out/bml9', '/SB/in/bml'
  c : Constant  Commented=on
  displayBMLs : MATLAB Function  TreatAsAtomicUnit=on
  increment_i : Subsystem  Commented=on
  makeBmls : MATLAB Function  TreatAsAtomicUnit=on
  wires:
  L/1 -> Scope/2, For Iterator/1, displayBMLs/2(l)
  AUs/1 -> makeBmls/2(arrAU)
  Amounts/1 -> makeBmls/3(eAmount)
  e1/1 -> displayBMLs/1(e)
  makeBmls/1(arrBML) -> Delay/1
  Unit Delay/1 -> Add/2
  c/1 -> Add/1
  Add/1 -> Unit Delay/1
  For Iterator/1 -> Scope/1, makeBmls/1(i), displayBMLs/3(i)
  Delay/1 -> displayBMLs/4(bml), bml1/1

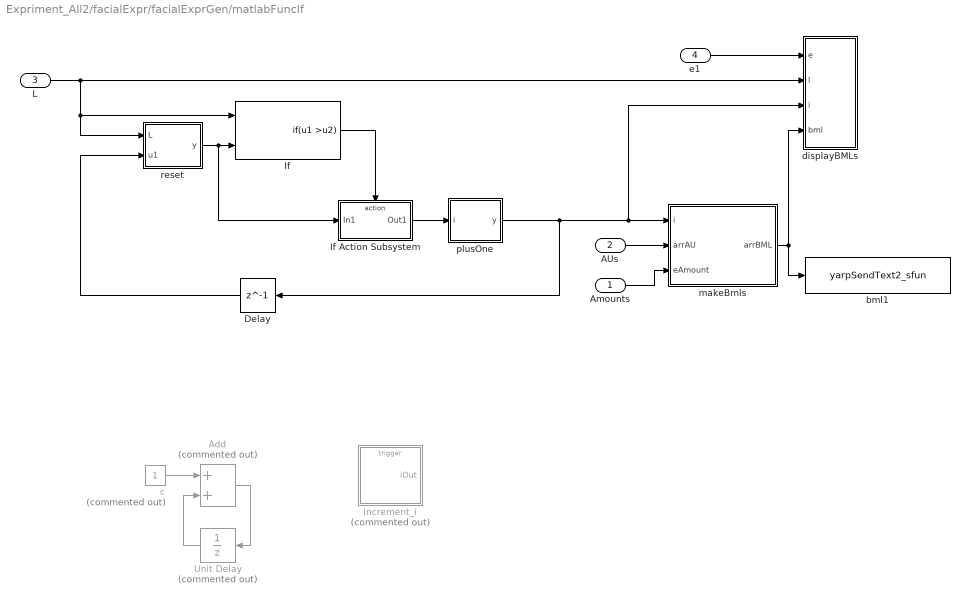
== system Expriment_All2/facialExpr/facialExprGen/matlabFuncIf ==
  Amounts : Inport
  AUs : Inport  Port=2
  L : Inport  Port=3
  e1 : Inport  Port=4
  Add : Sum  Commented=on
  Delay : Delay  DelayLength=1  InitialCondition=0
  If : If  NumInputs=2  IfExpression=u1 >u2  ShowElse=off
  If Action Subsystem : Subsystem  TreatAsAtomicUnit=on
  Unit Delay : UnitDelay  Commented=on  SampleTime=0.01
  bml1 : M-S-Function  FunctionName=yarpSendText2_sfun  Parameters='/sim/out/bml9', '/SB/in/bml'
  c : Constant  Commented=on
  displayBMLs : MATLAB Function  TreatAsAtomicUnit=on
  increment_i : Subsystem  Commented=on
  makeBmls : MATLAB Function  TreatAsAtomicUnit=on
  plusOne : MATLAB Function  TreatAsAtomicUnit=on
  reset : MATLAB Function  TreatAsAtomicUnit=on
  wires:
  L/1 -> reset/1(L), If/1, displayBMLs/2(l)
  AUs/1 -> makeBmls/2(arrAU)
  Amounts/1 -> makeBmls/3(eAmount)
  e1/1 -> displayBMLs/1(e)
  makeBmls/1(arrBML) -> displayBMLs/4(bml), bml1/1
  plusOne/1(y) -> Delay/1, displayBMLs/3(i), makeBmls/1(i)
  If/1 -> If Action Subsystem/Action
  Unit Delay/1 -> Add/2
  c/1 -> Add/1
  Add/1 -> Unit Delay/1
  If Action Subsystem/1(Out1) -> plusOne/1(i)
  Delay/1 -> reset/2(u1)
  reset/1(y) -> If Action Subsystem/1(In1), If/2

== system Expriment_All2/readGlove/normal glove/Normalize Index ==
  RawGlove : Inport
  Divide : Product  Inputs=*/  OutDataTypeStr=double  RndMeth=Nearest  InputSameDT=on
  Divide1 : Product  Inputs=**
  MinMax : Subsystem
  Range : Sum  Inputs=+-  OutDataTypeStr=double
  Ring1 : Constant  Value=100
  Subtract5 : Sum  Inputs=+-  OutDataTypeStr=double
  Norm100Out : Outport
  wires:
  MinMax/2(Max) -> Range/1
  Ring1/1 -> Divide1/2
  Subtract5/1 -> Divide/1
  MinMax/1(Min) -> Subtract5/2, Range/2
  RawGlove/1 -> Subtract5/1, MinMax/1(In1)
  Divide1/1 -> Norm100Out/1
  Divide/1 -> Divide1/1
  Range/1 -> Divide/2

== system Expriment_All2/readGlove/normal glove/Normalize Middle ==
  RawGlove : Inport
  Divide : Product  Inputs=*/  OutDataTypeStr=double  RndMeth=Nearest  InputSameDT=on
  Divide1 : Product  Inputs=**
  MinMax : Subsystem
  Range : Sum  Inputs=+-  OutDataTypeStr=double
  Ring1 : Constant  Value=100
  Subtract5 : Sum  Inputs=+-  OutDataTypeStr=double
  Norm100Out : Outport
  wires:
  MinMax/2(Max) -> Range/1
  Ring1/1 -> Divide1/2
  Subtract5/1 -> Divide/1
  MinMax/1(Min) -> Subtract5/2, Range/2
  RawGlove/1 -> Subtract5/1, MinMax/1(In1)
  Divide1/1 -> Norm100Out/1
  Divide/1 -> Divide1/1
  Range/1 -> Divide/2

== system Expriment_All2/readGlove/normal glove/Normalize Ring ==
  RawGlove : Inport
  Divide : Product  Inputs=*/  OutDataTypeStr=double  RndMeth=Nearest  InputSameDT=on
  Divide1 : Product  Inputs=**
  MinMax : Subsystem
  Range : Sum  Inputs=+-  OutDataTypeStr=double
  Ring1 : Constant  Value=100
  Subtract5 : Sum  Inputs=+-  OutDataTypeStr=double
  Norm100Out : Outport
  wires:
  MinMax/2(Max) -> Range/1
  Ring1/1 -> Divide1/2
  Subtract5/1 -> Divide/1
  MinMax/1(Min) -> Subtract5/2, Range/2
  RawGlove/1 -> Subtract5/1, MinMax/1(In1)
  Divide1/1 -> Norm100Out/1
  Divide/1 -> Divide1/1
  Range/1 -> Divide/2

== system Expriment_All2/facialExpr/facialExprGen/forloop/increment_i ==
  Trigger : TriggerPort  PortDimensions=1
  Add : Sum
  Scope : Scope  NumInputPorts=2
      settings: TimeRange=10  YMin=-5~-5  YMax=5~5  SaveName=ScopeData3
  Unit Delay : UnitDelay  SampleTime=0.01
  c : Constant
  iOut : Outport  OutMin=1  OutDataTypeStr=double  InitialOutput=1
  wires:
  Add/1 -> Scope/1, iOut/1, Unit Delay/1
  Unit Delay/1 -> Scope/2, Add/2
  c/1 -> Add/1

== system Expriment_All2/facialExpr/facialExprGen/forloop1/increment_i ==
  Trigger : TriggerPort  PortDimensions=1
  Add : Sum
  Scope : Scope  NumInputPorts=2
      settings: TimeRange=10  YMin=-5~-5  YMax=5~5  SaveName=ScopeData3
  Unit Delay : UnitDelay  SampleTime=0.01
  c : Constant
  iOut : Outport  OutMin=1  OutDataTypeStr=double  InitialOutput=1
  wires:
  Add/1 -> Scope/1, iOut/1, Unit Delay/1
  Unit Delay/1 -> Scope/2, Add/2
  c/1 -> Add/1

== system Expriment_All2/facialExpr/facialExprGen/matlabFuncIf/If Action Subsystem ==
  In1 : Inport
  Action Port : ActionPort  ActionType=then
  Scope : Scope
      settings: SaveName=ScopeData8
  Out1 : Outport
  wires:
  In1/1 -> Scope/1, Out1/1

== system Expriment_All2/facialExpr/facialExprGen/matlabFuncIf/increment_i ==
  Trigger : TriggerPort  PortDimensions=1
  Add : Sum
  Scope : Scope  NumInputPorts=2
      settings: TimeRange=10  YMin=-5~-5  YMax=5~5  SaveName=ScopeData3
  Unit Delay : UnitDelay  SampleTime=0.01
  c : Constant
  iOut : Outport  OutMin=1  OutDataTypeStr=double  InitialOutput=1
  wires:
  Add/1 -> Scope/1, iOut/1, Unit Delay/1
  Unit Delay/1 -> Scope/2, Add/2
  c/1 -> Add/1

== system Expriment_All2/readGlove/normal glove/Normalize Index/MinMax ==
  In1 : Inport
  Index1 : Constant  Value=0
  MinMax Running Resettable : simulink/Math Operations/MinMax Running Resettable  Function=min  vinit=100
  MinMax Running Resettable1 : simulink/Math Operations/MinMax Running Resettable  Function=max  vinit=0.0
  Min : Outport
  Max : Outport  Port=2
  wires:
  Index1/1 -> MinMax Running Resettable/2, MinMax Running Resettable1/2
  MinMax Running Resettable/1 -> Min/1
  In1/1 -> MinMax Running Resettable/1, MinMax Running Resettable1/1
  MinMax Running Resettable1/1 -> Max/1

== system Expriment_All2/readGlove/normal glove/Normalize Middle/MinMax ==
  In1 : Inport
  Index1 : Constant  Value=0
  MinMax Running Resettable : simulink/Math Operations/MinMax Running Resettable  Function=min  vinit=100
  MinMax Running Resettable1 : simulink/Math Operations/MinMax Running Resettable  Function=max  vinit=0.0
  Min : Outport
  Max : Outport  Port=2
  wires:
  Index1/1 -> MinMax Running Resettable/2, MinMax Running Resettable1/2
  MinMax Running Resettable/1 -> Min/1
  In1/1 -> MinMax Running Resettable/1, MinMax Running Resettable1/1
  MinMax Running Resettable1/1 -> Max/1

== system Expriment_All2/readGlove/normal glove/Normalize Ring/MinMax ==
  In1 : Inport
  Index1 : Constant  Value=0
  MinMax Running Resettable : simulink/Math Operations/MinMax Running Resettable  Function=min  vinit=100
  MinMax Running Resettable1 : simulink/Math Operations/MinMax Running Resettable  Function=max  vinit=0.0
  Min : Outport
  Max : Outport  Port=2
  wires:
  Index1/1 -> MinMax Running Resettable/2, MinMax Running Resettable1/2
  MinMax Running Resettable/1 -> Min/1
  In1/1 -> MinMax Running Resettable/1, MinMax Running Resettable1/1
  MinMax Running Resettable1/1 -> Max/1
